simulink model "PID"  (R2021a)
settings: Solver=VariableStepAuto  StartTime=0.0  StopTime=10.0  RelTol=1e-3
values from neighbouring files (symbols this model uses):
  den = [La*J (La*B + Ra*J) (Ra*B + Kb*K)]    [model_TF_motor_DC.m]
  num = K    (= 0.015)    [model_TF_motor_DC.m]
settings Model: Creator=Arya  LastModifiedBy=Arya

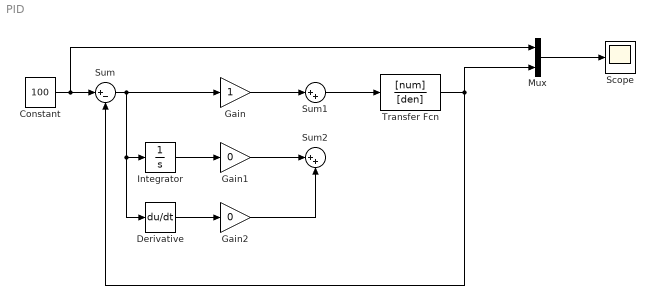
== system PID ==
  Constant : Constant  Value=100
  Derivative : Derivative
  Gain : Gain
  Gain1 : Gain  Gain=0
  Gain2 : Gain  Gain=0
  Integrator : Integrator
  Mux : Mux  Inputs=2
  Scope : Scope
  Sum : Sum  Inputs=|+-
  Sum1 : Sum  Inputs=|++
  Sum2 : Sum  Inputs=|++
  Transfer Fcn : TransferFcn  Numerator=[num]  Denominator=[den]
  wires:
  Constant/1 -> Mux/1, Sum/1
  Sum/1 -> Derivative/1, Integrator/1, Gain/1
  Integrator/1 -> Gain1/1
  Derivative/1 -> Gain2/1
  Gain1/1 -> Sum2/1
  Gain2/1 -> Sum2/2
  Gain/1 -> Sum1/1
  Sum1/1 -> Transfer Fcn/1
  Transfer Fcn/1 -> Mux/2, Sum/2
  Mux/1 -> Scope/1
